simulink model "singlcontact_control_smc_lqr_mydimes_reaction"  (R2024a)
settings: Solver=VariableStepAuto  StartTime=0.0  StopTime=10  FixedStep=0.001  RelTol=1e-3
values from neighbouring files (symbols this model uses):
  ankle_servo_kd = 8    [robotParametersCtrl_mydiem_block_zmp.m]    (also in robotParametersCtrl_quad_modify_mydiem.m; robotParametersCtrl_quad_modify_mydiem_reaction.m)
  ankle_servo_ki = 4    [robotParametersCtrl_mydiem_block_zmp.m]    (also in robotParametersCtrl_quad_modify_mydiem.m; robotParametersCtrl_quad_modify_mydiem_reaction.m)
  ankle_servo_kp = 20    [robotParametersCtrl_mydiem_block_zmp.m]    (also in robotParametersCtrl_quad_modify_mydiem.m; robotParametersCtrl_quad_modify_mydiem_reaction.m)
  deriv_filter_coeff = 100    [robotParametersCtrl_mydiem_block_zmp.m]    (also in robotParametersCtrl_quad_modify_mydiem.m; robotParametersCtrl_quad_modify_mydiem_reaction.m)
  filter_coefficent_pid = 100    [robotParametersCtrl_mydiem_block_zmp.m]    (also in robotParametersCtrl_quad_modify_mydiem.m; robotParametersCtrl_quad_modify_mydiem_reaction.m)
  filter_coefficent_pids = 100    [robotParametersCtrl_quad_modify_mydiem_reaction.m]
  foot_z = 1.5    [robotParametersCtrl_mydiem_block_zmp.m]    (also in robotParametersCtrl_quad_modify_mydiem.m; robotParametersCtrl_quad_modify_mydiem_reaction.m)
  g = 9.81    [ABCDvalues_lqr_quad_mydime_reaction.m]    (also in robotParametersCtrl_mydiem_block_zmp.m = 9.80665; robotParametersCtrl_quad_modify_mydiem.m = 9.80665; robotParametersCtrl_quad_modify_mydiem_reaction.m = 9.80665)
  h = 32    [robotParametersCtrl_mydiem_block_zmp.m]    (also in robotParametersCtrl_quad_modify_mydiem.m; robotParametersCtrl_quad_modify_mydiem_reaction.m)
  height_plane = 0.025    [robotParametersCtrl_mydiem_block_zmp.m]    (also in robotParametersCtrl_quad_modify_mydiem.m; robotParametersCtrl_quad_modify_mydiem_reaction.m)
  hip_pitch_deriv = 20    [robotParametersCtrl_mydiem_block_zmp.m]    (also in robotParametersCtrl_quad_modify_mydiem.m = 200; robotParametersCtrl_quad_modify_mydiem_reaction.m = 200)
  hip_pitch_derivs = 200    [robotParametersCtrl_quad_modify_mydiem_reaction.m]
  hip_pitch_int = 0    [robotParametersCtrl_mydiem_block_zmp.m]    (also in robotParametersCtrl_quad_modify_mydiem.m = 150; robotParametersCtrl_quad_modify_mydiem_reaction.m = 150)
  hip_pitch_ints = 1500    [robotParametersCtrl_quad_modify_mydiem_reaction.m]
  hip_pitch_prop = 10    [robotParametersCtrl_mydiem_block_zmp.m]    (also in robotParametersCtrl_quad_modify_mydiem.m = 500; robotParametersCtrl_quad_modify_mydiem_reaction.m = 500)
  hip_pitch_props = 500    [robotParametersCtrl_quad_modify_mydiem_reaction.m]
  hip_roll_deriv = 28    [robotParametersCtrl_mydiem_block_zmp.m]    (also in robotParametersCtrl_quad_modify_mydiem.m = 280; robotParametersCtrl_quad_modify_mydiem_reaction.m = 280)
  hip_roll_derivs = 280    [robotParametersCtrl_quad_modify_mydiem_reaction.m]
  hip_roll_int = 0    [robotParametersCtrl_mydiem_block_zmp.m]    (also in robotParametersCtrl_quad_modify_mydiem.m = 180; robotParametersCtrl_quad_modify_mydiem_reaction.m = 180)
  hip_roll_ints = 180    [robotParametersCtrl_quad_modify_mydiem_reaction.m]
  hip_roll_prop = 10    [robotParametersCtrl_mydiem_block_zmp.m]    (also in robotParametersCtrl_quad_modify_mydiem.m = 300; robotParametersCtrl_quad_modify_mydiem_reaction.m = 300)
  hip_roll_props = 300    [robotParametersCtrl_quad_modify_mydiem_reaction.m]
  hip_servo_kd = 20    [robotParametersCtrl_mydiem_block_zmp.m]    (also in robotParametersCtrl_quad_modify_mydiem.m; robotParametersCtrl_quad_modify_mydiem_reaction.m)
  hip_servo_ki = 10    [robotParametersCtrl_mydiem_block_zmp.m]    (also in robotParametersCtrl_quad_modify_mydiem.m; robotParametersCtrl_quad_modify_mydiem_reaction.m)
  hip_servo_kp = 60    [robotParametersCtrl_mydiem_block_zmp.m]    (also in robotParametersCtrl_quad_modify_mydiem.m; robotParametersCtrl_quad_modify_mydiem_reaction.m)
  hip_smc_lamda = 85    [robotParametersCtrl_mydiem_block_zmp.m]    (also in robotParametersCtrl_quad_modify_mydiem.m; robotParametersCtrl_quad_modify_mydiem_reaction.m = 95)
  hip_smc_lamdas = 85    [robotParametersCtrl_quad_modify_mydiem_reaction.m]
  hip_smc_new = 25    [robotParametersCtrl_mydiem_block_zmp.m]    (also in robotParametersCtrl_quad_modify_mydiem.m; robotParametersCtrl_quad_modify_mydiem_reaction.m = 45)
  hip_smc_news = 25    [robotParametersCtrl_quad_modify_mydiem_reaction.m]
  init_angs_L = init_angs_R    [robotParametersCtrl_mydiem_block_zmp.m]    (also in robotParametersCtrl_quad_modify_mydiem.m; robotParametersCtrl_quad_modify_mydiem_reaction.m)
  init_angs_R = [0 -sum(init_angs) init_angs(2) 0 init_angs(1)]    [robotParametersCtrl_mydiem_block_zmp.m]    (also in robotParametersCtrl_quad_modify_mydiem.m; robotParametersCtrl_quad_modify_mydiem_reaction.m)
  init_height = h +                torso_z/2 + torso_offset_z + height_plane/2    (= 39.5125)    [robotParametersCtrl_mydiem_block_zmp.m]    (also in robotParametersCtrl_quad_modify_mydiem.m; robotParametersCtrl_quad_modify_mydiem_reaction.m)
  K = lqr(A, B, Q, R)    [ABCDvalues_lqr_quad_mydime_reaction.m]
  knee_pitch_deriv = 10    [robotParametersCtrl_mydiem_block_zmp.m]    (also in robotParametersCtrl_quad_modify_mydiem.m = 100; robotParametersCtrl_quad_modify_mydiem_reaction.m = 100)
  knee_pitch_derivs = 180    [robotParametersCtrl_quad_modify_mydiem_reaction.m]
  knee_pitch_int = 0    [robotParametersCtrl_mydiem_block_zmp.m]    (also in robotParametersCtrl_quad_modify_mydiem.m = 300; robotParametersCtrl_quad_modify_mydiem_reaction.m = 300)
  knee_pitch_ints = 7500    [robotParametersCtrl_quad_modify_mydiem_reaction.m]
  knee_pitch_prop = 10    [robotParametersCtrl_mydiem_block_zmp.m]    (also in robotParametersCtrl_quad_modify_mydiem.m = 400; robotParametersCtrl_quad_modify_mydiem_reaction.m = 400)
  knee_pitch_props = 1200    [robotParametersCtrl_quad_modify_mydiem_reaction.m]
  knee_servo_kd = 10    [robotParametersCtrl_mydiem_block_zmp.m]    (also in robotParametersCtrl_quad_modify_mydiem.m; robotParametersCtrl_quad_modify_mydiem_reaction.m)
  knee_servo_ki = 5    [robotParametersCtrl_mydiem_block_zmp.m]    (also in robotParametersCtrl_quad_modify_mydiem.m; robotParametersCtrl_quad_modify_mydiem_reaction.m)
  knee_servo_kp = 60    [robotParametersCtrl_mydiem_block_zmp.m]    (also in robotParametersCtrl_quad_modify_mydiem.m; robotParametersCtrl_quad_modify_mydiem_reaction.m)
  knee_smc_lamda = 140    [robotParametersCtrl_mydiem_block_zmp.m]    (also in robotParametersCtrl_quad_modify_mydiem.m; robotParametersCtrl_quad_modify_mydiem_reaction.m = 150)
  knee_smc_lamdas = 100    [robotParametersCtrl_quad_modify_mydiem_reaction.m]
  knee_smc_new = 80    [robotParametersCtrl_mydiem_block_zmp.m]    (also in robotParametersCtrl_quad_modify_mydiem.m; robotParametersCtrl_quad_modify_mydiem_reaction.m)
  knee_smc_news = 60    [robotParametersCtrl_quad_modify_mydiem_reaction.m]
  Kwalk = 0.6    [robotParametersCtrl_mydiem_block_zmp.m]    (also in robotParametersCtrl_quad_modify_mydiem.m; robotParametersCtrl_quad_modify_mydiem_reaction.m)
  l1 = 0.20    (= 0.2)    [ABCDvalues_lqr_quad_mydime_reaction.m]
  l2 = 0.20    (= 0.2)    [ABCDvalues_lqr_quad_mydime_reaction.m]
  lower_leg_length = 20    [robotParametersCtrl_mydiem_block_zmp.m]    (also in robotParametersCtrl_quad_modify_mydiem.m; robotParametersCtrl_quad_modify_mydiem_reaction.m)
  m1 = 0.45    [ABCDvalues_lqr_quad_mydime_reaction.m]
  m2 = 0.065    [ABCDvalues_lqr_quad_mydime_reaction.m]
  max_torque = 20    [robotParametersCtrl_mydiem_block_zmp.m]    (also in robotParametersCtrl_quad_modify_mydiem.m; robotParametersCtrl_quad_modify_mydiem_reaction.m)
  motion_time_constant = 0.01    [robotParametersCtrl_mydiem_block_zmp.m]    (also in robotParametersCtrl_quad_modify_mydiem.m; robotParametersCtrl_quad_modify_mydiem_reaction.m)
  plane_x = 25    [robotParametersCtrl_mydiem_block_zmp.m]    (also in robotParametersCtrl_quad_modify_mydiem.m; robotParametersCtrl_quad_modify_mydiem_reaction.m)
  plane_y = 3    [robotParametersCtrl_mydiem_block_zmp.m]    (also in robotParametersCtrl_quad_modify_mydiem.m; robotParametersCtrl_quad_modify_mydiem_reaction.m)
  stepHeight = 0.4    [ABCDvalues_lqr_quad_mydime_reaction.m]
  torso_offset_x = 17    [robotParametersCtrl_mydiem_block_zmp.m]    (also in robotParametersCtrl_quad_modify_mydiem.m; robotParametersCtrl_quad_modify_mydiem_reaction.m)
  torso_offset_x1 = -17    [robotParametersCtrl_mydiem_block_zmp.m]    (also in robotParametersCtrl_quad_modify_mydiem.m; robotParametersCtrl_quad_modify_mydiem_reaction.m)
  torso_offset_z = 0    [robotParametersCtrl_mydiem_block_zmp.m]    (also in robotParametersCtrl_quad_modify_mydiem.m; robotParametersCtrl_quad_modify_mydiem_reaction.m)
  torso_x = 40    [robotParametersCtrl_mydiem_block_zmp.m]    (also in robotParametersCtrl_quad_modify_mydiem.m; robotParametersCtrl_quad_modify_mydiem_reaction.m)
  torso_y = 20    [robotParametersCtrl_mydiem_block_zmp.m]    (also in robotParametersCtrl_quad_modify_mydiem.m; robotParametersCtrl_quad_modify_mydiem_reaction.m)
  torso_z = 15    [robotParametersCtrl_mydiem_block_zmp.m]    (also in robotParametersCtrl_quad_modify_mydiem.m; robotParametersCtrl_quad_modify_mydiem_reaction.m)
  Ts = 0.05    [ABCDvalues_lqr_quad_mydime_reaction.m]
  TsCtrl = 0.05    [robotParametersCtrl_mydiem_block_zmp.m]    (also in robotParametersCtrl_quad_modify_mydiem.m; robotParametersCtrl_quad_modify_mydiem_reaction.m)
  tWalk = 0.3    [robotParametersCtrl_mydiem_block_zmp.m]    (also in robotParametersCtrl_quad_modify_mydiem.m; robotParametersCtrl_quad_modify_mydiem_reaction.m)
  upper_leg_length = 20    [robotParametersCtrl_mydiem_block_zmp.m]    (also in robotParametersCtrl_quad_modify_mydiem.m; robotParametersCtrl_quad_modify_mydiem_reaction.m)
undefined symbols (not defined in the file or in its folder): X, Y, Z
libraries: simulink_extras x256, slpidlib x128, sm_lib x71, simulink x43, nesl_utility x35, walkingRobotUtils x21, dspsrcs4 x18, dspobslib x8
(part 5 of 33)

== system singlcontact_control_smc_lqr_mydimes_reaction/Walking Robot/Lqr+Lqr+reaction/SMC Controllers FR3 ==
  ref : Inport
  meas : Inport  Port=2
  Bus Creator : BusCreator  Inputs=3
  Bus Selector : BusSelector  OutputSignals=knee_angle,hip_roll_angle,hip_pitch_angle
  Demux : Demux  Outputs=3
  Demux1 : Demux  Outputs=2
  Equivalent control : Subsystem
  Low-Pass Filter2 : simulink_extras/Additional Linear/Transfer Fcn (with initial outputs)  N=[(1/motion_time_constant)^2]  D=[1 2/motion_time_constant (1/motion_time_constant)^2]  Y0=init_angs_R(3)  U0=init_angs_R(3)
  Low-Pass Filter3 : simulink_extras/Additional Linear/Transfer Fcn (with initial outputs)  N=[(1/motion_time_constant)^2]  D=[1 2/motion_time_constant (1/motion_time_constant)^2]  Y0=init_angs_R(4)  U0=init_angs_R(4)
  Low-Pass Filter4 : simulink_extras/Additional Linear/Transfer Fcn (with initial outputs)  N=[(1/motion_time_constant)^2]  D=[1 2/motion_time_constant (1/motion_time_constant)^2]  Y0=init_angs_R(5)  U0=init_angs_R(5)
  Memory{,1..3} (4 alike) : Memory
  PID Hip Roll : slpidlib/PID Controller  Controller=PID  Form=Parallel  TimeDomain=Continuous-time  UseExternalTs=off  SampleTime=-1  IntegratorMethod=Forward Euler  FilterMethod=Forward Euler  ControllerParametersSource=internal  P=hip_servo_kp  I=hip_servo_ki  UseKiTs=off  D=hip_servo_kd  N=deriv_filter_coeff  UseFilter=on  TunerSelectOption=Transfer Function Based (PID Tuner App)  ZeroCross=off  InitialConditionSource=internal  InitialConditionForIntegrator=0  InitialConditionForFilter=0  DifferentiatorICPrevScaledInput=0  ExternalReset=none  TrackingMode=off  Kt=1  LimitOutput=on  SatLimitsSource=internal  UpperSaturationLimit=max_torque  LowerSaturationLimit=-max_torque  LinearizeAsGain=on  AntiWindupMode=clamping  Kb=1  LimitIntegrator=off  UpperIntegratorSaturationLimit=inf  LowerIntegratorSaturationLimit=-inf  POutMin=[]  POutMax=[]  IOutMin=[]  IOutMax=[]  DOutMin=[]  DOutMax=[]  NOutMin=[]  NOutMax=[]  SumOutMin=[]  SumOutMax=[]  SaturationOutMin=[]  SaturationOutMax=[]  PParamMin=[]  PParamMax=[]  IParamMin=[]  IParamMax=[]  DParamMin=[]  DParamMax=[]  NParamMin=[]  NParamMax=[]  KbParamMin=[]  KbParamMax=[]  KtParamMin=[]  KtParamMax=[]  KbOutMin=[]  KbOutMax=[]  KtOutMin=[]  KtOutMax=[]  IntegratorOutMin=[]  IntegratorOutMax=[]  FilterOutMin=[]  FilterOutMax=[]  SumI1OutMin=[]  SumI1OutMax=[]  SumI2OutMin=[]  SumI2OutMax=[]  SumI3OutMin=[]  SumI3OutMax=[]  SumI4OutMin=[]  SumI4OutMax=[]  SumDOutMin=[]  SumDOutMax=[]  DifferentiatorOutMin=[]  DifferentiatorOutMax=[]  FilterDiffOutCoefMin=[]  FilterDiffOutCoefMax=[]  ReciprocalOutMin=[]  ReciprocalOutMax=[]  SumDenOutMin=[]  SumDenOutMax=[]  SumNumOutMin=[]  SumNumOutMax=[]  DivideOutMin=[]  DivideOutMax=[]  UdiffTsProdOutMin=[]  UdiffTsProdOutMax=[]  NTsProdOutMin=[]  NTsProdOutMax=[]  UintegralTsProdOutMin=[]  UintegralTsProdOutMax=[]  UngainTsProdOutMin=[]  UngainTsProdOutMax=[]  ClampingZeroOutDataTypeStr=Inherit: Inherit via back propagation  ClampingZeroOutMin=[]  ClampingZeroOutMax=[]  FilterDenConstantOutDataTypeStr=Inherit: Inherit via back propagation  FilterDenConstantOutMin=[]  FilterDenConstantOutMax=[]  PCopyOutDataTypeStr=Inherit: Inherit via back propagation  PCopyOutMin=[]  PCopyOutMax=[]  NCopyOutDataTypeStr=Inherit: Inherit via back propagation  NCopyOutMin=[]  NCopyOutMax=[]  IntegratorContinuousStateAttributes=''  IntegratorStateMustResolveToSignalObject=off  IntegratorRTWStateStorageClass=Auto  FilterContinuousStateAttributes=''  FilterStateMustResolveToSignalObject=off  FilterRTWStateStorageClass=Auto  ParallelPVariant=InternalParameters  IdealPVariant=Disabled  IVariant=InternalParameters  DVariant=InternalParameters  IntegratorVariant=Continuous  SatVariant=Enabled  AWVariant=ContClampingParallel  PCopyVariant=Disabled  TRVariant=Disabled  FdbkBlocksVariant=Forward  IdealPFdbkVariant=Disabled  SatFdbkVariant=Disabled  DerivativeFilterVariant=ContFilter  NVariant=InternalParameters  NCopyVariant=Disabled  FilterICVariant=InternalICsFilter  IntegratorICVariant=InternalICs  ExternalResetVariant=Disabled  TRSumVariant=Passthrough  SumFdbkVariant=Disabled  SumVariant=Sum_PID  TsampFilterVariant=InternalTs  TsampNgainVariant=Passthrough  TsampIntegralVariant=Disabled_SignalSpec  ExternalSaturationOutDataTypeStr=Inherit: Same as second input
  SMC : Subsystem
  Sum2 : Sum  Inputs=|+-
  Sum3 : Sum  Inputs=|+-
  Sum7 : Sum  Inputs=|+-
  Input : Outport  VectorParamsAs1DForOutWhenUnconnected=off
  wires:
  Demux1/2 -> Bus Creator/3
  Demux1/1 -> Bus Creator/1
  SMC/1(Out1) -> Demux1/1
  Memory3/1 -> Equivalent control/3(theta2ddot)
  Memory2/1 -> Equivalent control/6(theta1ddot)
  Memory1/1 -> Equivalent control/4(theta1dot), Memory2/1
  Memory/1 -> Memory3/1, Equivalent control/5(theta2dot)
  meas/1 -> Bus Selector/1
  Bus Selector/2 -> Sum3/2  "<hip_roll_angle>"
  Low-Pass Filter4/1 -> Sum7/1
  Low-Pass Filter2/1 -> Sum2/1
  Bus Creator/1 -> Input/1
  Bus Selector/3 -> Sum7/2  "<hip_pitch_angle>"
  PID Hip Roll/1 -> Bus Creator/2  "hip roll"
  Low-Pass Filter3/1 -> Sum3/1
  Sum2/1 -> SMC/1(In1), Equivalent control/2(theta1), Memory1/1
  ref/1 -> Demux/1
  Sum3/1 -> PID Hip Roll/1
  Sum7/1 -> SMC/2(In2), Equivalent control/1(theta2), Memory/1
  Bus Selector/1 -> Sum2/2  "<knee_angle>"
  Demux/1 -> Low-Pass Filter2/1
  Demux/2 -> Low-Pass Filter3/1
  Demux/3 -> Low-Pass Filter4/1

== system singlcontact_control_smc_lqr_mydimes_reaction/Walking Robot/Lqr+Lqr+reaction/smc ==
  In1 : Inport
  Enable : EnablePort
  Out1 : Outport
  wires:
  In1/1 -> Out1/1

== system singlcontact_control_smc_lqr_mydimes_reaction/Walking Robot/Pid+Pid+reaction1/Lqr ==
  In1 : Inport
  Enable : EnablePort
  Out1 : Outport
  wires:
  In1/1 -> Out1/1

== system singlcontact_control_smc_lqr_mydimes_reaction/Walking Robot/Pid+Pid+reaction1/PID Controllers FR ==
  ref : Inport
  meas : Inport  Port=2
  Bus Creator : BusCreator  Inputs=3
  Bus Selector : BusSelector  OutputSignals=knee_angle,hip_roll_angle,hip_pitch_angle
  Demux : Demux  Outputs=3
  Low-Pass Filter2 : simulink_extras/Additional Linear/Transfer Fcn (with initial outputs)  N=[(1/motion_time_constant)^2]  D=[1 2/motion_time_constant (1/motion_time_constant)^2]  Y0=init_angs_R(3)  U0=init_angs_R(3)
  Low-Pass Filter3 : simulink_extras/Additional Linear/Transfer Fcn (with initial outputs)  N=[(1/motion_time_constant)^2]  D=[1 2/motion_time_constant (1/motion_time_constant)^2]  Y0=init_angs_R(4)  U0=init_angs_R(4)
  Low-Pass Filter4 : simulink_extras/Additional Linear/Transfer Fcn (with initial outputs)  N=[(1/motion_time_constant)^2]  D=[1 2/motion_time_constant (1/motion_time_constant)^2]  Y0=init_angs_R(5)  U0=init_angs_R(5)
  Mux : Mux  Inputs=2
  Mux1 : Mux  Inputs=2
  Mux2 : Mux  Inputs=2
  PID Hip Roll : slpidlib/PID Controller  Controller=PID  Form=Parallel  TimeDomain=Continuous-time  UseExternalTs=off  SampleTime=-1  IntegratorMethod=Forward Euler  FilterMethod=Forward Euler  ControllerParametersSource=internal  P=hip_roll_prop  I=hip_roll_int  UseKiTs=off  D=hip_roll_deriv  N=deriv_filter_coeff  UseFilter=on  TunerSelectOption=Transfer Function Based (PID Tuner App)  ZeroCross=off  InitialConditionSource=internal  InitialConditionForIntegrator=0  InitialConditionForFilter=0  DifferentiatorICPrevScaledInput=0  ExternalReset=none  TrackingMode=off  Kt=1  LimitOutput=on  SatLimitsSource=internal  UpperSaturationLimit=max_torque  LowerSaturationLimit=-max_torque  LinearizeAsGain=on  AntiWindupMode=clamping  Kb=1  LimitIntegrator=off  UpperIntegratorSaturationLimit=inf  LowerIntegratorSaturationLimit=-inf  POutMin=[]  POutMax=[]  IOutMin=[]  IOutMax=[]  DOutMin=[]  DOutMax=[]  NOutMin=[]  NOutMax=[]  SumOutMin=[]  SumOutMax=[]  SaturationOutMin=[]  SaturationOutMax=[]  PParamMin=[]  PParamMax=[]  IParamMin=[]  IParamMax=[]  DParamMin=[]  DParamMax=[]  NParamMin=[]  NParamMax=[]  KbParamMin=[]  KbParamMax=[]  KtParamMin=[]  KtParamMax=[]  KbOutMin=[]  KbOutMax=[]  KtOutMin=[]  KtOutMax=[]  IntegratorOutMin=[]  IntegratorOutMax=[]  FilterOutMin=[]  FilterOutMax=[]  SumI1OutMin=[]  SumI1OutMax=[]  SumI2OutMin=[]  SumI2OutMax=[]  SumI3OutMin=[]  SumI3OutMax=[]  SumI4OutMin=[]  SumI4OutMax=[]  SumDOutMin=[]  SumDOutMax=[]  DifferentiatorOutMin=[]  DifferentiatorOutMax=[]  FilterDiffOutCoefMin=[]  FilterDiffOutCoefMax=[]  ReciprocalOutMin=[]  ReciprocalOutMax=[]  SumDenOutMin=[]  SumDenOutMax=[]  SumNumOutMin=[]  SumNumOutMax=[]  DivideOutMin=[]  DivideOutMax=[]  UdiffTsProdOutMin=[]  UdiffTsProdOutMax=[]  NTsProdOutMin=[]  NTsProdOutMax=[]  UintegralTsProdOutMin=[]  UintegralTsProdOutMax=[]  UngainTsProdOutMin=[]  UngainTsProdOutMax=[]  ClampingZeroOutDataTypeStr=Inherit: Inherit via back propagation  ClampingZeroOutMin=[]  ClampingZeroOutMax=[]  FilterDenConstantOutDataTypeStr=Inherit: Inherit via back propagation  FilterDenConstantOutMin=[]  FilterDenConstantOutMax=[]  PCopyOutDataTypeStr=Inherit: Inherit via back propagation  PCopyOutMin=[]  PCopyOutMax=[]  NCopyOutDataTypeStr=Inherit: Inherit via back propagation  NCopyOutMin=[]  NCopyOutMax=[]  IntegratorContinuousStateAttributes=''  IntegratorStateMustResolveToSignalObject=off  IntegratorRTWStateStorageClass=Auto  FilterContinuousStateAttributes=''  FilterStateMustResolveToSignalObject=off  FilterRTWStateStorageClass=Auto  ParallelPVariant=InternalParameters  IdealPVariant=Disabled  IVariant=InternalParameters  DVariant=InternalParameters  IntegratorVariant=Continuous  SatVariant=Enabled  AWVariant=ContClampingParallel  PCopyVariant=Disabled  TRVariant=Disabled  FdbkBlocksVariant=Forward  IdealPFdbkVariant=Disabled  SatFdbkVariant=Disabled  DerivativeFilterVariant=ContFilter  NVariant=InternalParameters  NCopyVariant=Disabled  FilterICVariant=InternalICsFilter  IntegratorICVariant=InternalICs  ExternalResetVariant=Disabled  TRSumVariant=Passthrough  SumFdbkVariant=Disabled  SumVariant=Sum_PID  TsampFilterVariant=InternalTs  TsampNgainVariant=Passthrough  TsampIntegralVariant=Disabled_SignalSpec  ExternalSaturationOutDataTypeStr=Inherit: Same as second input
  PID Hip pitch : slpidlib/PID Controller  Controller=PID  Form=Parallel  TimeDomain=Continuous-time  UseExternalTs=off  SampleTime=-1  IntegratorMethod=Forward Euler  FilterMethod=Forward Euler  ControllerParametersSource=internal  P=hip_pitch_prop  I=hip_pitch_int  UseKiTs=off  D=hip_pitch_deriv  N=deriv_filter_coeff  UseFilter=on  TunerSelectOption=Transfer Function Based (PID Tuner App)  ZeroCross=off  InitialConditionSource=internal  InitialConditionForIntegrator=0  InitialConditionForFilter=0  DifferentiatorICPrevScaledInput=0  ExternalReset=none  TrackingMode=off  Kt=1  LimitOutput=on  SatLimitsSource=internal  UpperSaturationLimit=max_torque  LowerSaturationLimit=-max_torque  LinearizeAsGain=on  AntiWindupMode=clamping  Kb=1  LimitIntegrator=off  UpperIntegratorSaturationLimit=inf  LowerIntegratorSaturationLimit=-inf  POutMin=[]  POutMax=[]  IOutMin=[]  IOutMax=[]  DOutMin=[]  DOutMax=[]  NOutMin=[]  NOutMax=[]  SumOutMin=[]  SumOutMax=[]  SaturationOutMin=[]  SaturationOutMax=[]  PParamMin=[]  PParamMax=[]  IParamMin=[]  IParamMax=[]  DParamMin=[]  DParamMax=[]  NParamMin=[]  NParamMax=[]  KbParamMin=[]  KbParamMax=[]  KtParamMin=[]  KtParamMax=[]  KbOutMin=[]  KbOutMax=[]  KtOutMin=[]  KtOutMax=[]  IntegratorOutMin=[]  IntegratorOutMax=[]  FilterOutMin=[]  FilterOutMax=[]  SumI1OutMin=[]  SumI1OutMax=[]  SumI2OutMin=[]  SumI2OutMax=[]  SumI3OutMin=[]  SumI3OutMax=[]  SumI4OutMin=[]  SumI4OutMax=[]  SumDOutMin=[]  SumDOutMax=[]  DifferentiatorOutMin=[]  DifferentiatorOutMax=[]  FilterDiffOutCoefMin=[]  FilterDiffOutCoefMax=[]  ReciprocalOutMin=[]  ReciprocalOutMax=[]  SumDenOutMin=[]  SumDenOutMax=[]  SumNumOutMin=[]  SumNumOutMax=[]  DivideOutMin=[]  DivideOutMax=[]  UdiffTsProdOutMin=[]  UdiffTsProdOutMax=[]  NTsProdOutMin=[]  NTsProdOutMax=[]  UintegralTsProdOutMin=[]  UintegralTsProdOutMax=[]  UngainTsProdOutMin=[]  UngainTsProdOutMax=[]  ClampingZeroOutDataTypeStr=Inherit: Inherit via back propagation  ClampingZeroOutMin=[]  ClampingZeroOutMax=[]  FilterDenConstantOutDataTypeStr=Inherit: Inherit via back propagation  FilterDenConstantOutMin=[]  FilterDenConstantOutMax=[]  PCopyOutDataTypeStr=Inherit: Inherit via back propagation  PCopyOutMin=[]  PCopyOutMax=[]  NCopyOutDataTypeStr=Inherit: Inherit via back propagation  NCopyOutMin=[]  NCopyOutMax=[]  IntegratorContinuousStateAttributes=''  IntegratorStateMustResolveToSignalObject=off  IntegratorRTWStateStorageClass=Auto  FilterContinuousStateAttributes=''  FilterStateMustResolveToSignalObject=off  FilterRTWStateStorageClass=Auto  ParallelPVariant=InternalParameters  IdealPVariant=Disabled  IVariant=InternalParameters  DVariant=InternalParameters  IntegratorVariant=Continuous  SatVariant=Enabled  AWVariant=ContClampingParallel  PCopyVariant=Disabled  TRVariant=Disabled  FdbkBlocksVariant=Forward  IdealPFdbkVariant=Disabled  SatFdbkVariant=Disabled  DerivativeFilterVariant=ContFilter  NVariant=InternalParameters  NCopyVariant=Disabled  FilterICVariant=InternalICsFilter  IntegratorICVariant=InternalICs  ExternalResetVariant=Disabled  TRSumVariant=Passthrough  SumFdbkVariant=Disabled  SumVariant=Sum_PID  TsampFilterVariant=InternalTs  TsampNgainVariant=Passthrough  TsampIntegralVariant=Disabled_SignalSpec  ExternalSaturationOutDataTypeStr=Inherit: Same as second input
  PID knee : slpidlib/PID Controller  Controller=PID  Form=Parallel  TimeDomain=Continuous-time  UseExternalTs=off  SampleTime=-1  IntegratorMethod=Forward Euler  FilterMethod=Forward Euler  ControllerParametersSource=internal  P=knee_pitch_prop  I=knee_pitch_int  UseKiTs=off  D=knee_pitch_deriv  N=deriv_filter_coeff  UseFilter=on  TunerSelectOption=Transfer Function Based (PID Tuner App)  ZeroCross=off  InitialConditionSource=internal  InitialConditionForIntegrator=0  InitialConditionForFilter=0  DifferentiatorICPrevScaledInput=0  ExternalReset=none  TrackingMode=off  Kt=1  LimitOutput=on  SatLimitsSource=internal  UpperSaturationLimit=max_torque  LowerSaturationLimit=-max_torque  LinearizeAsGain=on  AntiWindupMode=clamping  Kb=1  LimitIntegrator=off  UpperIntegratorSaturationLimit=inf  LowerIntegratorSaturationLimit=-inf  POutMin=[]  POutMax=[]  IOutMin=[]  IOutMax=[]  DOutMin=[]  DOutMax=[]  NOutMin=[]  NOutMax=[]  SumOutMin=[]  SumOutMax=[]  SaturationOutMin=[]  SaturationOutMax=[]  PParamMin=[]  PParamMax=[]  IParamMin=[]  IParamMax=[]  DParamMin=[]  DParamMax=[]  NParamMin=[]  NParamMax=[]  KbParamMin=[]  KbParamMax=[]  KtParamMin=[]  KtParamMax=[]  KbOutMin=[]  KbOutMax=[]  KtOutMin=[]  KtOutMax=[]  IntegratorOutMin=[]  IntegratorOutMax=[]  FilterOutMin=[]  FilterOutMax=[]  SumI1OutMin=[]  SumI1OutMax=[]  SumI2OutMin=[]  SumI2OutMax=[]  SumI3OutMin=[]  SumI3OutMax=[]  SumI4OutMin=[]  SumI4OutMax=[]  SumDOutMin=[]  SumDOutMax=[]  DifferentiatorOutMin=[]  DifferentiatorOutMax=[]  FilterDiffOutCoefMin=[]  FilterDiffOutCoefMax=[]  ReciprocalOutMin=[]  ReciprocalOutMax=[]  SumDenOutMin=[]  SumDenOutMax=[]  SumNumOutMin=[]  SumNumOutMax=[]  DivideOutMin=[]  DivideOutMax=[]  UdiffTsProdOutMin=[]  UdiffTsProdOutMax=[]  NTsProdOutMin=[]  NTsProdOutMax=[]  UintegralTsProdOutMin=[]  UintegralTsProdOutMax=[]  UngainTsProdOutMin=[]  UngainTsProdOutMax=[]  ClampingZeroOutDataTypeStr=Inherit: Inherit via back propagation  ClampingZeroOutMin=[]  ClampingZeroOutMax=[]  FilterDenConstantOutDataTypeStr=Inherit: Inherit via back propagation  FilterDenConstantOutMin=[]  FilterDenConstantOutMax=[]  PCopyOutDataTypeStr=Inherit: Inherit via back propagation  PCopyOutMin=[]  PCopyOutMax=[]  NCopyOutDataTypeStr=Inherit: Inherit via back propagation  NCopyOutMin=[]  NCopyOutMax=[]  IntegratorContinuousStateAttributes=''  IntegratorStateMustResolveToSignalObject=off  IntegratorRTWStateStorageClass=Auto  FilterContinuousStateAttributes=''  FilterStateMustResolveToSignalObject=off  FilterRTWStateStorageClass=Auto  ParallelPVariant=InternalParameters  IdealPVariant=Disabled  IVariant=InternalParameters  DVariant=InternalParameters  IntegratorVariant=Continuous  SatVariant=Enabled  AWVariant=ContClampingParallel  PCopyVariant=Disabled  TRVariant=Disabled  FdbkBlocksVariant=Forward  IdealPFdbkVariant=Disabled  SatFdbkVariant=Disabled  DerivativeFilterVariant=ContFilter  NVariant=InternalParameters  NCopyVariant=Disabled  FilterICVariant=InternalICsFilter  IntegratorICVariant=InternalICs  ExternalResetVariant=Disabled  TRSumVariant=Passthrough  SumFdbkVariant=Disabled  SumVariant=Sum_PID  TsampFilterVariant=InternalTs  TsampNgainVariant=Passthrough  TsampIntegralVariant=Disabled_SignalSpec  ExternalSaturationOutDataTypeStr=Inherit: Same as second input
  Scope : Scope
  Scope1 : Scope  NumInputPorts=3
  Sum2 : Sum  Inputs=|+-
  Sum3 : Sum  Inputs=|+-
  Sum7 : Sum  Inputs=|+-
  Input : Outport  VectorParamsAs1DForOutWhenUnconnected=off
  wires:
  meas/1 -> Bus Selector/1
  Bus Selector/2 -> Mux1/2, Sum3/2  "<hip_roll_angle>"
  Bus Creator/1 -> Scope/1, Input/1
  PID Hip Roll/1 -> Bus Creator/2  "hip roll"
  Low-Pass Filter3/1 -> Mux1/1, Sum3/1
  Sum2/1 -> PID knee/1
  ref/1 -> Demux/1
  Demux/1 -> Low-Pass Filter2/1
  Demux/2 -> Low-Pass Filter3/1
  Demux/3 -> Low-Pass Filter4/1
  PID knee/1 -> Bus Creator/1  "knee"
  PID Hip pitch/1 -> Bus Creator/3  "hip pitch"
  Sum7/1 -> PID Hip pitch/1
  Sum3/1 -> PID Hip Roll/1
  Mux1/1 -> Scope1/2
  Mux/1 -> Scope1/1
  Mux2/1 -> Scope1/3
  Low-Pass Filter2/1 -> Mux/1, Sum2/1
  Bus Selector/1 -> Mux/2, Sum2/2  "<knee_angle>"
  Low-Pass Filter4/1 -> Mux2/1, Sum7/1
  Bus Selector/3 -> Mux2/2, Sum7/2  "<hip_pitch_angle>"

== system singlcontact_control_smc_lqr_mydimes_reaction/Walking Robot/Pid+Pid+reaction1/PID Controllers FR1 ==
  ref : Inport
  meas : Inport  Port=2
  Bus Creator : BusCreator  Inputs=3
  Bus Selector : BusSelector  OutputSignals=knee_angle,hip_roll_angle,hip_pitch_angle
  Demux : Demux  Outputs=3
  Low-Pass Filter2 : simulink_extras/Additional Linear/Transfer Fcn (with initial outputs)  N=[(1/motion_time_constant)^2]  D=[1 2/motion_time_constant (1/motion_time_constant)^2]  Y0=init_angs_R(3)  U0=init_angs_R(3)
  Low-Pass Filter3 : simulink_extras/Additional Linear/Transfer Fcn (with initial outputs)  N=[(1/motion_time_constant)^2]  D=[1 2/motion_time_constant (1/motion_time_constant)^2]  Y0=init_angs_R(4)  U0=init_angs_R(4)
  Low-Pass Filter4 : simulink_extras/Additional Linear/Transfer Fcn (with initial outputs)  N=[(1/motion_time_constant)^2]  D=[1 2/motion_time_constant (1/motion_time_constant)^2]  Y0=init_angs_R(5)  U0=init_angs_R(5)
  PID Hip Roll : slpidlib/PID Controller  Controller=PID  Form=Parallel  TimeDomain=Continuous-time  UseExternalTs=off  SampleTime=-1  IntegratorMethod=Forward Euler  FilterMethod=Forward Euler  ControllerParametersSource=internal  P=hip_roll_prop  I=hip_roll_int  UseKiTs=off  D=hip_roll_deriv  N=deriv_filter_coeff  UseFilter=on  TunerSelectOption=Transfer Function Based (PID Tuner App)  ZeroCross=off  InitialConditionSource=internal  InitialConditionForIntegrator=0  InitialConditionForFilter=0  DifferentiatorICPrevScaledInput=0  ExternalReset=none  TrackingMode=off  Kt=1  LimitOutput=on  SatLimitsSource=internal  UpperSaturationLimit=max_torque  LowerSaturationLimit=-max_torque  LinearizeAsGain=on  AntiWindupMode=clamping  Kb=1  LimitIntegrator=off  UpperIntegratorSaturationLimit=inf  LowerIntegratorSaturationLimit=-inf  POutMin=[]  POutMax=[]  IOutMin=[]  IOutMax=[]  DOutMin=[]  DOutMax=[]  NOutMin=[]  NOutMax=[]  SumOutMin=[]  SumOutMax=[]  SaturationOutMin=[]  SaturationOutMax=[]  PParamMin=[]  PParamMax=[]  IParamMin=[]  IParamMax=[]  DParamMin=[]  DParamMax=[]  NParamMin=[]  NParamMax=[]  KbParamMin=[]  KbParamMax=[]  KtParamMin=[]  KtParamMax=[]  KbOutMin=[]  KbOutMax=[]  KtOutMin=[]  KtOutMax=[]  IntegratorOutMin=[]  IntegratorOutMax=[]  FilterOutMin=[]  FilterOutMax=[]  SumI1OutMin=[]  SumI1OutMax=[]  SumI2OutMin=[]  SumI2OutMax=[]  SumI3OutMin=[]  SumI3OutMax=[]  SumI4OutMin=[]  SumI4OutMax=[]  SumDOutMin=[]  SumDOutMax=[]  DifferentiatorOutMin=[]  DifferentiatorOutMax=[]  FilterDiffOutCoefMin=[]  FilterDiffOutCoefMax=[]  ReciprocalOutMin=[]  ReciprocalOutMax=[]  SumDenOutMin=[]  SumDenOutMax=[]  SumNumOutMin=[]  SumNumOutMax=[]  DivideOutMin=[]  DivideOutMax=[]  UdiffTsProdOutMin=[]  UdiffTsProdOutMax=[]  NTsProdOutMin=[]  NTsProdOutMax=[]  UintegralTsProdOutMin=[]  UintegralTsProdOutMax=[]  UngainTsProdOutMin=[]  UngainTsProdOutMax=[]  ClampingZeroOutDataTypeStr=Inherit: Inherit via back propagation  ClampingZeroOutMin=[]  ClampingZeroOutMax=[]  FilterDenConstantOutDataTypeStr=Inherit: Inherit via back propagation  FilterDenConstantOutMin=[]  FilterDenConstantOutMax=[]  PCopyOutDataTypeStr=Inherit: Inherit via back propagation  PCopyOutMin=[]  PCopyOutMax=[]  NCopyOutDataTypeStr=Inherit: Inherit via back propagation  NCopyOutMin=[]  NCopyOutMax=[]  IntegratorContinuousStateAttributes=''  IntegratorStateMustResolveToSignalObject=off  IntegratorRTWStateStorageClass=Auto  FilterContinuousStateAttributes=''  FilterStateMustResolveToSignalObject=off  FilterRTWStateStorageClass=Auto  ParallelPVariant=InternalParameters  IdealPVariant=Disabled  IVariant=InternalParameters  DVariant=InternalParameters  IntegratorVariant=Continuous  SatVariant=Enabled  AWVariant=ContClampingParallel  PCopyVariant=Disabled  TRVariant=Disabled  FdbkBlocksVariant=Forward  IdealPFdbkVariant=Disabled  SatFdbkVariant=Disabled  DerivativeFilterVariant=ContFilter  NVariant=InternalParameters  NCopyVariant=Disabled  FilterICVariant=InternalICsFilter  IntegratorICVariant=InternalICs  ExternalResetVariant=Disabled  TRSumVariant=Passthrough  SumFdbkVariant=Disabled  SumVariant=Sum_PID  TsampFilterVariant=InternalTs  TsampNgainVariant=Passthrough  TsampIntegralVariant=Disabled_SignalSpec  ExternalSaturationOutDataTypeStr=Inherit: Same as second input
  PID Hip pitch : slpidlib/PID Controller  Controller=PID  Form=Parallel  TimeDomain=Continuous-time  UseExternalTs=off  SampleTime=-1  IntegratorMethod=Forward Euler  FilterMethod=Forward Euler  ControllerParametersSource=internal  P=hip_pitch_prop  I=hip_pitch_int  UseKiTs=off  D=hip_pitch_deriv  N=deriv_filter_coeff  UseFilter=on  TunerSelectOption=Transfer Function Based (PID Tuner App)  ZeroCross=off  InitialConditionSource=internal  InitialConditionForIntegrator=0  InitialConditionForFilter=0  DifferentiatorICPrevScaledInput=0  ExternalReset=none  TrackingMode=off  Kt=1  LimitOutput=on  SatLimitsSource=internal  UpperSaturationLimit=max_torque  LowerSaturationLimit=-max_torque  LinearizeAsGain=on  AntiWindupMode=clamping  Kb=1  LimitIntegrator=off  UpperIntegratorSaturationLimit=inf  LowerIntegratorSaturationLimit=-inf  POutMin=[]  POutMax=[]  IOutMin=[]  IOutMax=[]  DOutMin=[]  DOutMax=[]  NOutMin=[]  NOutMax=[]  SumOutMin=[]  SumOutMax=[]  SaturationOutMin=[]  SaturationOutMax=[]  PParamMin=[]  PParamMax=[]  IParamMin=[]  IParamMax=[]  DParamMin=[]  DParamMax=[]  NParamMin=[]  NParamMax=[]  KbParamMin=[]  KbParamMax=[]  KtParamMin=[]  KtParamMax=[]  KbOutMin=[]  KbOutMax=[]  KtOutMin=[]  KtOutMax=[]  IntegratorOutMin=[]  IntegratorOutMax=[]  FilterOutMin=[]  FilterOutMax=[]  SumI1OutMin=[]  SumI1OutMax=[]  SumI2OutMin=[]  SumI2OutMax=[]  SumI3OutMin=[]  SumI3OutMax=[]  SumI4OutMin=[]  SumI4OutMax=[]  SumDOutMin=[]  SumDOutMax=[]  DifferentiatorOutMin=[]  DifferentiatorOutMax=[]  FilterDiffOutCoefMin=[]  FilterDiffOutCoefMax=[]  ReciprocalOutMin=[]  ReciprocalOutMax=[]  SumDenOutMin=[]  SumDenOutMax=[]  SumNumOutMin=[]  SumNumOutMax=[]  DivideOutMin=[]  DivideOutMax=[]  UdiffTsProdOutMin=[]  UdiffTsProdOutMax=[]  NTsProdOutMin=[]  NTsProdOutMax=[]  UintegralTsProdOutMin=[]  UintegralTsProdOutMax=[]  UngainTsProdOutMin=[]  UngainTsProdOutMax=[]  ClampingZeroOutDataTypeStr=Inherit: Inherit via back propagation  ClampingZeroOutMin=[]  ClampingZeroOutMax=[]  FilterDenConstantOutDataTypeStr=Inherit: Inherit via back propagation  FilterDenConstantOutMin=[]  FilterDenConstantOutMax=[]  PCopyOutDataTypeStr=Inherit: Inherit via back propagation  PCopyOutMin=[]  PCopyOutMax=[]  NCopyOutDataTypeStr=Inherit: Inherit via back propagation  NCopyOutMin=[]  NCopyOutMax=[]  IntegratorContinuousStateAttributes=''  IntegratorStateMustResolveToSignalObject=off  IntegratorRTWStateStorageClass=Auto  FilterContinuousStateAttributes=''  FilterStateMustResolveToSignalObject=off  FilterRTWStateStorageClass=Auto  ParallelPVariant=InternalParameters  IdealPVariant=Disabled  IVariant=InternalParameters  DVariant=InternalParameters  IntegratorVariant=Continuous  SatVariant=Enabled  AWVariant=ContClampingParallel  PCopyVariant=Disabled  TRVariant=Disabled  FdbkBlocksVariant=Forward  IdealPFdbkVariant=Disabled  SatFdbkVariant=Disabled  DerivativeFilterVariant=ContFilter  NVariant=InternalParameters  NCopyVariant=Disabled  FilterICVariant=InternalICsFilter  IntegratorICVariant=InternalICs  ExternalResetVariant=Disabled  TRSumVariant=Passthrough  SumFdbkVariant=Disabled  SumVariant=Sum_PID  TsampFilterVariant=InternalTs  TsampNgainVariant=Passthrough  TsampIntegralVariant=Disabled_SignalSpec  ExternalSaturationOutDataTypeStr=Inherit: Same as second input
  PID knee : slpidlib/PID Controller  Controller=PID  Form=Parallel  TimeDomain=Continuous-time  UseExternalTs=off  SampleTime=-1  IntegratorMethod=Forward Euler  FilterMethod=Forward Euler  ControllerParametersSource=internal  P=knee_pitch_prop  I=knee_pitch_int  UseKiTs=off  D=knee_pitch_deriv  N=deriv_filter_coeff  UseFilter=on  TunerSelectOption=Transfer Function Based (PID Tuner App)  ZeroCross=off  InitialConditionSource=internal  InitialConditionForIntegrator=0  InitialConditionForFilter=0  DifferentiatorICPrevScaledInput=0  ExternalReset=none  TrackingMode=off  Kt=1  LimitOutput=on  SatLimitsSource=internal  UpperSaturationLimit=max_torque  LowerSaturationLimit=-max_torque  LinearizeAsGain=on  AntiWindupMode=clamping  Kb=1  LimitIntegrator=off  UpperIntegratorSaturationLimit=inf  LowerIntegratorSaturationLimit=-inf  POutMin=[]  POutMax=[]  IOutMin=[]  IOutMax=[]  DOutMin=[]  DOutMax=[]  NOutMin=[]  NOutMax=[]  SumOutMin=[]  SumOutMax=[]  SaturationOutMin=[]  SaturationOutMax=[]  PParamMin=[]  PParamMax=[]  IParamMin=[]  IParamMax=[]  DParamMin=[]  DParamMax=[]  NParamMin=[]  NParamMax=[]  KbParamMin=[]  KbParamMax=[]  KtParamMin=[]  KtParamMax=[]  KbOutMin=[]  KbOutMax=[]  KtOutMin=[]  KtOutMax=[]  IntegratorOutMin=[]  IntegratorOutMax=[]  FilterOutMin=[]  FilterOutMax=[]  SumI1OutMin=[]  SumI1OutMax=[]  SumI2OutMin=[]  SumI2OutMax=[]  SumI3OutMin=[]  SumI3OutMax=[]  SumI4OutMin=[]  SumI4OutMax=[]  SumDOutMin=[]  SumDOutMax=[]  DifferentiatorOutMin=[]  DifferentiatorOutMax=[]  FilterDiffOutCoefMin=[]  FilterDiffOutCoefMax=[]  ReciprocalOutMin=[]  ReciprocalOutMax=[]  SumDenOutMin=[]  SumDenOutMax=[]  SumNumOutMin=[]  SumNumOutMax=[]  DivideOutMin=[]  DivideOutMax=[]  UdiffTsProdOutMin=[]  UdiffTsProdOutMax=[]  NTsProdOutMin=[]  NTsProdOutMax=[]  UintegralTsProdOutMin=[]  UintegralTsProdOutMax=[]  UngainTsProdOutMin=[]  UngainTsProdOutMax=[]  ClampingZeroOutDataTypeStr=Inherit: Inherit via back propagation  ClampingZeroOutMin=[]  ClampingZeroOutMax=[]  FilterDenConstantOutDataTypeStr=Inherit: Inherit via back propagation  FilterDenConstantOutMin=[]  FilterDenConstantOutMax=[]  PCopyOutDataTypeStr=Inherit: Inherit via back propagation  PCopyOutMin=[]  PCopyOutMax=[]  NCopyOutDataTypeStr=Inherit: Inherit via back propagation  NCopyOutMin=[]  NCopyOutMax=[]  IntegratorContinuousStateAttributes=''  IntegratorStateMustResolveToSignalObject=off  IntegratorRTWStateStorageClass=Auto  FilterContinuousStateAttributes=''  FilterStateMustResolveToSignalObject=off  FilterRTWStateStorageClass=Auto  ParallelPVariant=InternalParameters  IdealPVariant=Disabled  IVariant=InternalParameters  DVariant=InternalParameters  IntegratorVariant=Continuous  SatVariant=Enabled  AWVariant=ContClampingParallel  PCopyVariant=Disabled  TRVariant=Disabled  FdbkBlocksVariant=Forward  IdealPFdbkVariant=Disabled  SatFdbkVariant=Disabled  DerivativeFilterVariant=ContFilter  NVariant=InternalParameters  NCopyVariant=Disabled  FilterICVariant=InternalICsFilter  IntegratorICVariant=InternalICs  ExternalResetVariant=Disabled  TRSumVariant=Passthrough  SumFdbkVariant=Disabled  SumVariant=Sum_PID  TsampFilterVariant=InternalTs  TsampNgainVariant=Passthrough  TsampIntegralVariant=Disabled_SignalSpec  ExternalSaturationOutDataTypeStr=Inherit: Same as second input
  Scope : Scope
  Sum2 : Sum  Inputs=|+-
  Sum3 : Sum  Inputs=|+-
  Sum7 : Sum  Inputs=|+-
  Input : Outport  VectorParamsAs1DForOutWhenUnconnected=off
  wires:
  meas/1 -> Bus Selector/1
  Bus Selector/2 -> Sum3/2  "<hip_roll_angle>"
  Bus Creator/1 -> Scope/1, Input/1
  PID Hip Roll/1 -> Bus Creator/2  "hip roll"
  Low-Pass Filter3/1 -> Sum3/1
  Sum2/1 -> PID knee/1
  ref/1 -> Demux/1
  Demux/1 -> Low-Pass Filter2/1
  Demux/2 -> Low-Pass Filter3/1
  Demux/3 -> Low-Pass Filter4/1
  PID knee/1 -> Bus Creator/1  "knee"
  PID Hip pitch/1 -> Bus Creator/3  "hip pitch"
  Sum7/1 -> PID Hip pitch/1
  Sum3/1 -> PID Hip Roll/1
  Low-Pass Filter2/1 -> Sum2/1
  Bus Selector/1 -> Sum2/2  "<knee_angle>"
  Low-Pass Filter4/1 -> Sum7/1
  Bus Selector/3 -> Sum7/2  "<hip_pitch_angle>"
